simulink model "motor_io_position_GABRIEL"  (R2014b)
settings: Solver=ode1  StartTime=0.0  StopTime=inf  FixedStep=Ts  RelTol=1e-3
PostLoadFcn:
  | , if any(exist('dsrtsu_mdlpostloadfcn', 'file') == [2, 3, 6]), try dsrtsu_mdlpostloadfcn('Execute', bdroot); catch fprintf('Error in PostLoadFcn (dsrtsu_mdlpostloadfcn) for model "%s":\n %s\n', bdroot, lasterr); end, end,
values from neighbouring files (symbols this model uses):
  F_c = 1.5e-3    (= 0.0015)    [continuous_design.m]    (also in workshop1.m)
  F_c_lower = 1.5e-3    (= 0.0015)    [continuous_design.m]    (also in workshop1.m)
  F_c_upper = 1.5e-3    (= 0.0015)    [continuous_design.m]    (also in workshop1.m)
  J1 = 0.0006    [continuous_design.m]    (also in workshop1.m)
  motor = motor_pars    [continuous_design.m]    (also in workshop1.m)
  n = 5    [continuous_design.m]    (also in workshop1.m)
  R_sim = Rd.num{1}    [pbutest.m]
  S_sim = Sd.num{1}    [pbutest.m]
  T_sim = Td.num{1}    [pbutest.m]
  Ts = 2*pi/ws    (= 0.0199466200228)    [continuous_design.m]    (also in pbutest.m = 0.0108705628152; workshop1.m = Ts_p)
libraries: rtilib1104 x5, simulink x1
settings Model: DSRTSU_INTERNAL_RTI_VER=450  DSRTSU_INTERNAL_RTI_TYPE=rti1104  DSRTSU_INTERNAL_RTIFPGA=40  ExtModeArmWhenConnect=off  BufferReuse=off  Creator=user  LastModifiedBy=es2lab2
settings DataIOCC: SignalLoggingSaveFormat=ModelDataLogs  SaveOutput=off  SignalLoggingName=sigsOut
settings OptimizationCC: BlockReduction=off  ConditionallyExecuteInputs=off  OptimizeBlockIOStorage=off  BufferReuse=off  GlobalBufferReuse=off  ExpressionFolding=off  ExpressionDepthLimit=2147483647  LocalBlockOutputs=off  InitFltsAndDblsToZero=on
settings DebuggingCC: SaveWithParameterizedLinksMsg=none  UnderspecifiedInitializationDetection=Classic  MergeDetectMultiDrivingBlocksExec=none  SignalResolutionControl=TryResolveAllWithWarning  SolverPrmCheckMsg=none  MultiTaskDSMMsg=warning  MultiTaskCondExecSysMsg=none  FcnCallInpInsideContextMsg=UseLocalSettings  UnconnectedInputMsg=none  UnconnectedOutputMsg=none  StateNameClashWarn=warning
settings HardwareCC: ProdIntDivRoundTo=Zero  ProdEndianess=BigEndian  ProdHWDeviceType=Generic->Custom  TargetIntDivRoundTo=Zero  TargetEndianess=BigEndian  TargetHWDeviceType=Generic->Custom
settings RTWCC: SystemTargetFile=rti1104.tlc  MakeCommand=make_rti  TemplateMakefile=rti1104.tmf  Description=dSPACE DS1104 Hardware Platform  RetainRTWFile=on  ProcessScript=rti1104_make_rtw_hook  IncludeERTFirstTime=on
settings STFCustomTargetCC: TargetFcnLib=ansi_tfl_tmw.mat  ParMdlRefBuildCompliant=on  GeneratePreprocessorConditionals=Disable all  SystemTargetFile=rti1104.tlc
settings GRTTargetCC: TargetFcnLib=ansi_tfl_tmw.mat  CompOptLevelCompliant=off  ConcurrentExecutionCompliant=off  CombineOutputUpdateFcns=off  MatFileLogging=off  CPPClassGenCompliant=off  GRTInterface=on  ExtModeMexFile=noextcomm

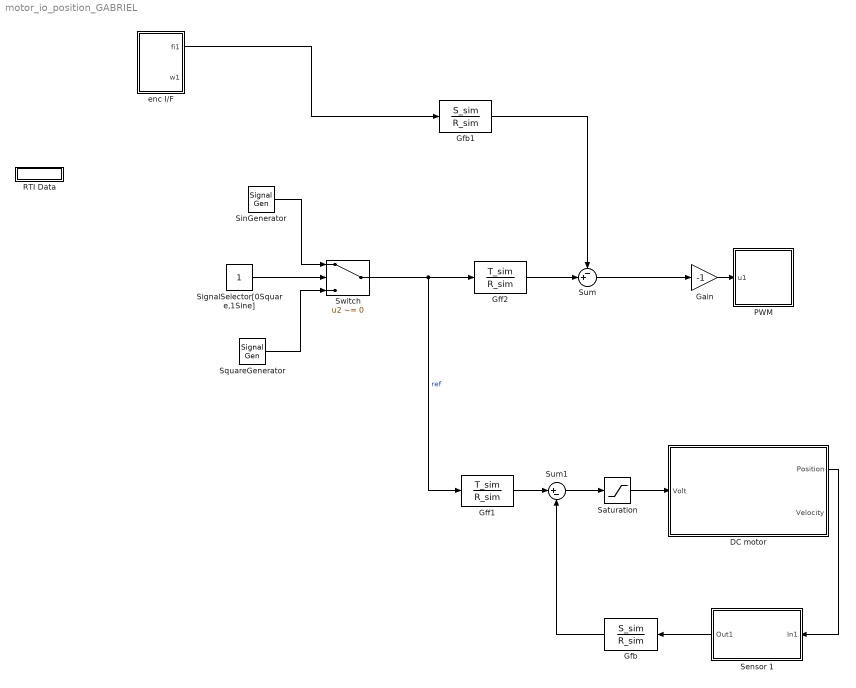
== system motor_io_position_GABRIEL ==
  DC motor : Subsystem
  Gain : Gain  Gain=-1
  Gfb : DiscreteTransferFcn  Numerator=S_sim  Denominator=R_sim  SampleTime=Ts
  Gfb1 : DiscreteTransferFcn  Numerator=S_sim  Denominator=R_sim  SampleTime=Ts
  Gff1 : DiscreteTransferFcn  Numerator=T_sim  Denominator=R_sim  SampleTime=Ts
  Gff2 : DiscreteTransferFcn  Numerator=T_sim  Denominator=R_sim  SampleTime=Ts
  PWM : Subsystem
  RTI Data : Subsystem  Tag=struct('RTIDataServer',struct('RTIDataServerVs','2','RTIModelDescription','struct(''main'',''motor_io_position_GABRIEL'',''sub'',''motor_io_position_GABRIEL'',''isMp'',0)'))  LoadFcn="if exist('rtidc'), try,  rtidc('DataHostBlockClbLoad', gcbh); catch, disp(['Warning: ''LoadFcn'' for RTI Data block failed: ' lasterr]); end, end,"  mask(RTI_DATA_HOST){}
      mask help:
      | RTI Data Block.
      | This block is used by RTI to store internal model-dependent data.
      | Please keep this block on the root level of the model. Deleting this block will result in data loss.
      |
      | NEVER DELETE OR COPY THIS BLOCK!
      settings: CopyFcn="if exist('rtidc'), try,  rtidc('DataHostBlockClbCopy', gcbh); catch, disp(['Warning: ''CopyFcn'' for RTI Data block failed: ' lasterr]); end, end,"  DeleteFcn="if exist('rtidc'), try,  rtidc('DataHostBlockClbDelete', gcbh); catch, disp(['Warning: ''DeleteFcn'' for RTI Data block failed: ' lasterr]); end, end,"  ModelCloseFcn="if exist('rtidc'), try,  rtidc('DataHostBlockClbModelClose', gcbh); catch, disp(['Warning: ''ModelCloseFcn'' for RTI Data block failed: ' lasterr]); end, end,"  PreSaveFcn="if exist('rtidc'), try,  rtidc('DataHostBlockClbPreSave', gcbh); catch, disp(['Warning: ''PreSaveFcn'' for RTI Data block failed: ' lasterr]); end, end,"  PostSaveFcn="if exist('rtidc'), try,  rtidc('DataHostBlockClbPostSave', gcbh); catch, disp(['Warning: ''PostSaveFcn'' for RTI Data block failed: ' lasterr]); end, end,"  NameChangeFcn="if exist('rtidc'), try,  rtidc('DataHostBlockClbNameChange', gcbh); catch, disp(['Warning: ''NameChangeFcn'' for RTI Data block failed: ' lasterr]); end, end,"
      mask Help:
      | RTI Data Block.
      | This block is used by RTI to store internal model-dependent data.
      | Please keep this block on the root level of the model. Deleting this block will result in data loss.
      | 
      | NEVER DELETE OR COPY THIS BLOCK!
      mask Display:
      | text(0.5, 0.5, 'RTI Data', 'HorizontalAlignment', 'center');
      | plot([1 0]);
  Saturation : Saturate  UpperLimit=24  LowerLimit=-24
  Sensor 1 : Subsystem
  SignalSelector[0Square,1Sine] : Constant
  SinGenerator : SignalGenerator  Amplitude=0  Units=rad/sec
  SquareGenerator : SignalGenerator  WaveForm=square  Amplitude=0  Units=rad/sec
  Sum : Sum  Inputs=-+|
  Sum1 : Sum  Inputs=|+-
  Switch : Switch  Criteria=u2 ~= 0
  enc I/F : Subsystem
  wires:
  SinGenerator/1 -> Switch/1
  SquareGenerator/1 -> Switch/3
  SignalSelector[0Square,1Sine]/1 -> Switch/2
  Switch/1 -> Gff1/1, Gff2/1  "ref"
  ? -> ?
  Gain/1 -> PWM/1(u1)
  enc I/F/1(fi1) -> Gfb1/1
  Gfb1/1 -> Sum/1
  Gff2/1 -> Sum/2
  Sum/1 -> Gain/1
  Sensor 1/1(Out1) -> Gfb/1
  DC motor/1(Position) -> Sensor 1/1(In1)
  Saturation/1 -> DC motor/1(Volt)
  Gfb/1 -> Sum1/2
  Sum1/1 -> Saturation/1
  Gff1/1 -> Sum1/1

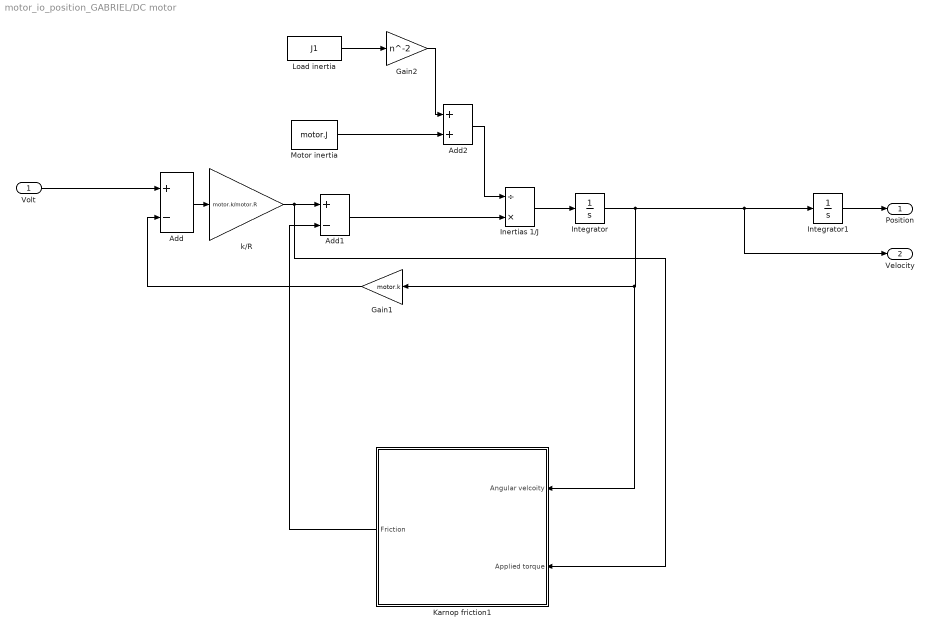
== system motor_io_position_GABRIEL/DC motor ==
  Volt : Inport
  Add : Sum  Inputs=+-
  Add1 : Sum  Inputs=+-
  Add2 : Sum
  Gain1 : Gain  Gain=motor.k
  Gain2 : Gain  Gain=n^-2
  Inertias 1/J : Product  Inputs=/*
  Integrator : Integrator
  Integrator1 : Integrator
  Karnop friction1 : Subsystem
  Load inertia : Constant  Value=J1
  Motor inertia : Constant  Value=motor.J
  "k/R " : Gain  Gain=motor.k/motor.R
  Position : Outport
  Velocity : Outport  Port=2
  wires:
  Add2/1 -> Inertias 1/J/1
  Gain2/1 -> Add2/1
  Load inertia/1 -> Gain2/1
  Motor inertia/1 -> Add2/2
  Integrator/1 -> Integrator1/1, Velocity/1, Gain1/1, Karnop friction1/1(Angular velcoity)
  Volt/1 -> Add/1
  Add1/1 -> Inertias 1/J/2
  Integrator1/1 -> Position/1
  Inertias 1/J/1 -> Integrator/1
  "k/R "/1 -> Add1/1, Karnop friction1/2(Applied torque)
  Add/1 -> "k/R "/1
  Gain1/1 -> Add/2
  Karnop friction1/1(Friction) -> Add1/2

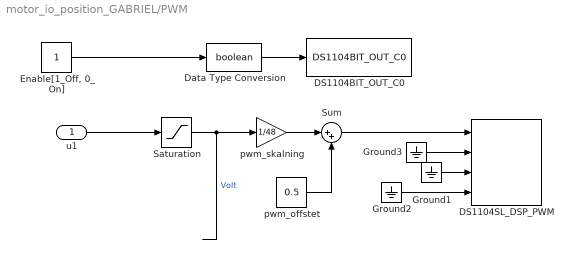
== system motor_io_position_GABRIEL/PWM ==
  u1 : Inport
  DS1104BIT_OUT_C0 : rtilib1104/DS1104 MASTER PPC/DS1104BIT_OUT_C0  ChannelNo=0  InitValue=1  TermMode=0  TermValue=0  Reserved1=[]  Reserved2=[]  Reserved3=[]  Reserved=[]  DialogFcn=gui1104bit_out  UnitName={'DS1104BIT_OUT_C'}  UnitValues={ 0 }  DSProperties=struct('RTI',struct('Version',uint32(1),'BlockType',struct('isSLSource',uint8(0),'isSLSink',uint8(1),'isHWSource',uint8(0),'isHWSink',uint8(1),'isSetup',uint8(0),'isInline',uint8(1),'isNonInline',uint8(0),'isInterrupt',uint8(0),'isChannelwise',uint8(1)),'IOBoardType','DS1104MASTER','UnitType','BIT','Identifier','BITOUTCH','DialogType','ML','BlockSet','NONE','SlaveProcessor','NONE'))
  DS1104SL_DSP_PWM : rtilib1104/DS1104 SLAVE DSP/DS1104SL_DSP_PWM  Parameters=[]  TDef=[]  BoardType=[]  PwmMode=1  Frequency=20000  InitValue=[0.5 0.5 0.5 0.5]  TermMode=[0 0 0 0]  TermValue=[0.5 0.5 0.5 0.5]  Polarity=[1 1 1 1]  DialogFcn=gui1104sl_dsp_pwm  Reserved1=[]  Reserved2=[]  Reserved3=[]  Reserved4=[]  Revision=[]  UnitName={'DS1104SL_DSP_PWM'}  UnitValues={[]}  DSProperties=struct('RTI',struct('Version',uint32(2),'BlockType',struct('isSLSource',uint8(0),'isSLSink',uint8(1),'isHWSource',uint8(0),'isHWSink',uint8(1),'isSetup',uint8(0),'isInline',uint8(1),'isNonInline',uint8(0),'isInterrupt',uint8(0),'isChannelwise',uint8(0)),'IOBoardType','DS1104SLAVE','UnitType','PWM','Identifier','PWM','DialogType','ML','BlockSet','NONE','SlaveProcessor','F240'))  RTIBlockInterface=struct('InputPortsActive',[1 1 1 1],'InputPortsWidth',int32([1 1 1 1]),'InputPortsName',{{['PWM Channel 1'],['PWM Channel 2'],['PWM Channel 3'],['PWM Channel 4']}},'IWork',{{{'',uint32(4)}}},'DialogFcn','rti1104slavepwmgui','InitLevel',1,'BlockDisplay',{{'','auto'}},'IconTransparency','on','MultiSFcn',4,'BlockName',struct('Token',{{'DS1104SL_DSP_PWM'}}))  RTIBlockParameters=struct('PWMSymmetryMode',{{1,'OFF',[]}},'PWMFrequency',{{'50000','OFF',[]}},'PWMPolarityMode',{{[1 1 1 1 1],'OFF',[]}},'ChannelNo',{{[1 2 3 4],'OFF',[]}},'SuspendModeInit',{{[0 0 0 0 1],'OFF',[]}},'TTLModeInit',{{[2 2 2 2 2],'OFF',[]}},'DutyCycleInitValueCh1',{{'0.5','OFF',[]}},'DutyCycleInitValueCh2',{{'0.5','OFF',[]}},'DutyCycleInitValueCh3',{{'0.5','OFF',[]}},'DutyCycleInitValueCh4',{{'0.5','OFF',[]}},'DutyCycleInitValueCh5',{{'0.5','OFF',[]}},'EnablePWMStop',{{[0 0 0 0 0],'OFF',[]}},'SuspendModeTerm',{{[0 0 0 0 1],'OFF',[]}},'TTLModeTerm',{{[2 2 2 2 2],'OFF',[]}},'DutyCycleTermValueCh1',{{'0.5','OFF',[]}},'DutyCycleTermValueCh2',{{'0.5','OFF',[]}},'DutyCycleTermValueCh3',{{'0.5','OFF',[]}},'DutyCycleTermValueCh4',{{'0.5','OFF',[]}},'DutyCycleTermValueCh5',{{'0.5','OFF',[]}},'TLCFileName',{{'rti1104pwm','OFF',[]}})  RTISFcnParameters=struct('PWMSymmetryMode','double','PWMFrequency','double','PWMPolarityMode','double','ChannelNo','double','SuspendModeInit','double','TTLModeInit','double','DutyCycleInitValueCh1','double','DutyCycleInitValueCh2','double','DutyCycleInitValueCh3','double','DutyCycleInitValueCh4','double','EnablePWMStop','double','SuspendModeTerm','double','TTLModeTerm','double','DutyCycleTermValueCh1','double','DutyCycleTermValueCh2','double','DutyCycleTermValueCh3','double','DutyCycleTermValueCh4','double','TLCFileName','char')  RTIBlockParaDefault=struct('PWMSymmetryMode',1,'PWMFrequency',100,'PWMPolarityMode',[1 1 1 1 1],'ChannelNo',[1 2 3 4],'SuspendModeInit',[1 1 1 1 1],'TTLModeInit',[2 2 2 2 2],'DutyCycleInitValueCh1',0.5,'DutyCycleInitValueCh2',0.5,'DutyCycleInitValueCh3',0.5,'DutyCycleInitValueCh4',0.5,'DutyCycleInitValueCh5',0.5,'EnablePWMStop',[1 1 1 1 0],'SuspendModeTerm',[1 1 1 1 1],'TTLModeTerm',[2 2 2 2 2],'DutyCycleTermValueCh1',0.5,'DutyCycleTermValueCh2',0.5,'DutyCycleTermValueCh3',0.5,'DutyCycleTermValueCh4',0.5,'DutyCycleTermValueCh5',0.5,'TLCFileName','rti1104pwm')
  Data Type Conversion : DataTypeConversion  OutDataTypeStr=boolean  SaturateOnIntegerOverflow=on  RndMeth=Zero
  "Enable[1_Off, 0_On]" : Constant
  Ground1 : Ground
  Ground2 : Ground
  Ground3 : Ground
  Saturation : Saturate  UpperLimit=24  LowerLimit=-24
  Sum : Sum  Inputs=|++  SaturateOnIntegerOverflow=on
  pwm_offstet : Constant  Value=0.5
  pwm_skalning : Gain  Gain=1/48  SaturateOnIntegerOverflow=on  OutDataTypeStr=Inherit: Same as input  ParamDataTypeStr=Inherit: Same as input
  wires:
  "Enable[1_Off, 0_On]"/1 -> Data Type Conversion/1
  Data Type Conversion/1 -> DS1104BIT_OUT_C0/1
  pwm_skalning/1 -> Sum/1
  Sum/1 -> DS1104SL_DSP_PWM/1
  pwm_offstet/1 -> Sum/2
  u1/1 -> Saturation/1
  Ground1/1 -> DS1104SL_DSP_PWM/3
  Ground2/1 -> DS1104SL_DSP_PWM/4
  Ground3/1 -> DS1104SL_DSP_PWM/2
  Saturation/1 -> pwm_skalning/1  "Volt"

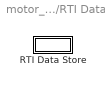
== system motor_io_position_GABRIEL/RTI Data ==
  RTI Data Store : Subsystem  Tag=struct('private',struct('version',struct('dsVer',uint32(2)),'access',struct('modified',['06-Apr-2016 18:22:15'],'type','Model','isPerm',1)))  mask(RTI_DATA_STORE){}
      mask help:
      | RTI Data Store Block. This block is used by RTI to store internal model dependent data. Deleting this block will result in data loss.
      |
      | NEVER DELETE, COPY, OR MODIFY THIS BLOCK!
      mask Help:
      | RTI Data Store Block. This block is used by RTI to store internal model dependent data. Deleting this block will result in data loss.
      | 
      | NEVER DELETE, COPY, OR MODIFY THIS BLOCK!
      mask Display: text(0.5, 0.5, ' ', 'HorizontalAlignment', 'center');

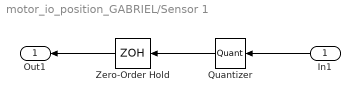
== system motor_io_position_GABRIEL/Sensor 1 ==
  In1 : Inport
  Quantizer : Quantizer  QuantizationInterval=quant
  Zero-Order Hold : ZeroOrderHold  SampleTime=Ts
  Out1 : Outport
  wires:
  Quantizer/1 -> Zero-Order Hold/1
  In1/1 -> Quantizer/1
  Zero-Order Hold/1 -> Out1/1

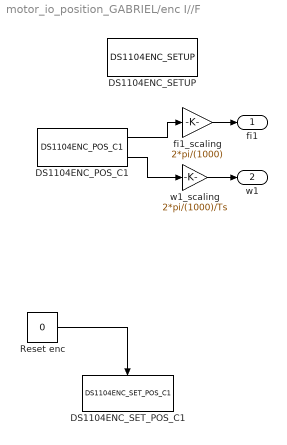
== system motor_io_position_GABRIEL/enc I//F ==
  DS1104ENC_POS_C1 : rtilib1104/DS1104 MASTER PPC/DS1104ENC_POS_C1  ChannelNo=1  PosValue=0  Reserved1=[]  Reserved2=[]  Reserved3=[]  Reserved4=[]  DialogFcn=gui1104enc_pos  UnitName={'DS1104ENC_POS_C'}  UnitValues={ 1 }  DSProperties=struct('RTI',struct('Version',uint32(1),'BlockType',struct('isSLSource',uint8(1),'isSLSink',uint8(0),'isHWSource',uint8(1),'isHWSink',uint8(0),'isSetup',uint8(0),'isInline',uint8(1),'isNonInline',uint8(0),'isInterrupt',uint8(0),'isChannelwise',uint8(1)),'IOBoardType','DS1104MASTER','UnitType','ENC','Identifier','ENCPOSCH','DialogType','ML','BlockSet','NONE','SlaveProcessor','NONE'))
  DS1104ENC_SETUP : rtilib1104/DS1104 MASTER PPC/DS1104ENC_SETUP  Reserved1=[]  Reserved2=[]  Reserved3=[]  Reserved4=[]  DialogFcn=gui1104enc_setup  UnitName={'DS1104ENC_SETUP'}  UnitValues={ [] }  DSProperties=struct('RTI',struct('Version',uint32(1),'BlockType',struct('isSLSource',uint8(0),'isSLSink',uint8(0),'isHWSource',uint8(0),'isHWSink',uint8(0),'isSetup',uint8(0),'isInline',uint8(1),'isNonInline',uint8(0),'isInterrupt',uint8(0),'isChannelwise',uint8(0)),'IOBoardType','DS1104MASTER','UnitType','ENC','Identifier','ENCSETUP','DialogType','ML','BlockSet','NONE','SlaveProcessor','NONE'))
      settings: SignalType=[1 0]
  DS1104ENC_SET_POS_C1 : rtilib1104/DS1104 MASTER PPC/DS1104ENC_SET_POS_C1  ChannelNo=1  PosValue=0  Reserved1=[]  Reserved2=[]  Reserved3=[]  Reserved4=[]  DialogFcn=gui1104enc_set_pos  UnitName={'DS1104ENC_SET_POS_C'}  UnitValues={ 1 }  DSProperties=struct('RTI',struct('Version',uint32(1),'BlockType',struct('isSLSource',uint8(0),'isSLSink',uint8(1),'isHWSource',uint8(0),'isHWSink',uint8(1),'isSetup',uint8(0),'isInline',uint8(1),'isNonInline',uint8(0),'isInterrupt',uint8(0),'isChannelwise',uint8(1)),'IOBoardType','DS1104MASTER','UnitType','ENC','Identifier','ENCRESET','DialogType','ML','BlockSet','NONE','SlaveProcessor','NONE'))
  Reset enc : Constant  Value=0
  fi1_scaling : Gain  Gain=2*pi/(1000)  SaturateOnIntegerOverflow=on  OutDataTypeStr=Inherit: Same as input  ParamDataTypeStr=Inherit: Same as input
  w1_scaling : Gain  Gain=2*pi/(1000)/Ts  SaturateOnIntegerOverflow=on  OutDataTypeStr=Inherit: Same as input  ParamDataTypeStr=Inherit: Same as input
  fi1 : Outport
  w1 : Outport  Port=2
  wires:
  Reset enc/1 -> DS1104ENC_SET_POS_C1/Trigger
  DS1104ENC_POS_C1/1 -> fi1_scaling/1
  DS1104ENC_POS_C1/2 -> w1_scaling/1
  fi1_scaling/1 -> fi1/1
  w1_scaling/1 -> w1/1

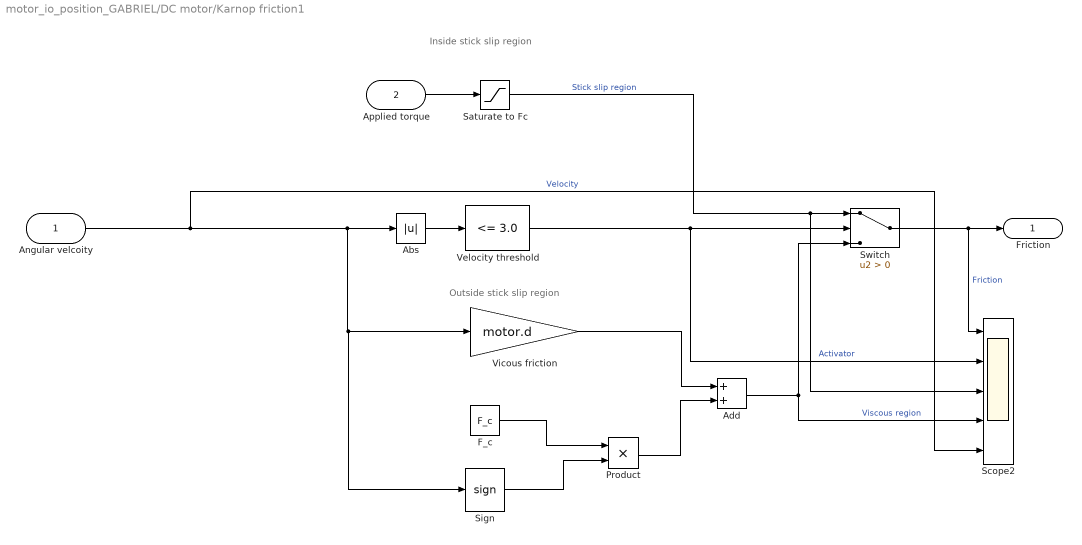
== system motor_io_position_GABRIEL/DC motor/Karnop friction1 ==
  note: Outside stick slip region
  note: Inside stick slip region
  Angular velcoity : Inport
  Applied torque : Inport  Port=2
  Abs : Abs  ZeroCross=off
  Add : Sum
  F_c : Constant  Value=F_c
  Product : Product
  Saturate to Fc : Saturate  UpperLimit=F_c_upper  LowerLimit=-F_c_lower  ZeroCross=off
  Scope2 : Scope  NumInputPorts=5
      settings: ShowLegends=on  YMin=-0.00177~-0.125~0.0009~-0.00177~-138.1533~-0.12501~-0.12501~-0.12501  YMax=0.00177~1.125~0.0011~0.00177~138.10681~0.12501~0.12501~0.12501  SaveName=ScopeData3
  Sign : Signum  ZeroCross=off
  Switch : Switch  Criteria=u2 > Threshold  ZeroCross=off
  "Velocity threshold " : simulink/Logic and Bit Operations/Compare To Constant  relop=<=  const=3.0  OutDataTypeStr=boolean
  Vicous friction : Gain  Gain=motor.d
  Friction : Outport
  wires:
  Applied torque/1 -> Saturate to Fc/1
  Add/1 -> Scope2/4, Switch/3  "Viscous region"
  Sign/1 -> Product/2
  F_c/1 -> Product/1
  Vicous friction/1 -> Add/1
  Product/1 -> Add/2
  Abs/1 -> "Velocity threshold "/1
  "Velocity threshold "/1 -> Switch/2, Scope2/2  "Activator"
  Angular velcoity/1 -> Sign/1, Vicous friction/1, Abs/1, Scope2/5  "Velocity"
  Switch/1 -> Friction/1, Scope2/1  "Friction"
  Saturate to Fc/1 -> Switch/1, Scope2/3  "Stick slip region"

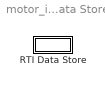
== system motor_io_position_GABRIEL/RTI Data/RTI Data Store ==
  RTI Data Store : Subsystem  mask(RTI_DATA_STORE){}
      mask help:
      | RTI Data Store Block. This block is used by RTI to store internal model dependent data. Deleting this block will result in data loss.
      |
      | NEVER DELETE, COPY, OR MODIFY THIS BLOCK!
      mask Help:
      | RTI Data Store Block. This block is used by RTI to store internal model dependent data. Deleting this block will result in data loss.
      | 
      | NEVER DELETE, COPY, OR MODIFY THIS BLOCK!
      mask Display: text(0.5, 0.5, ' ', 'HorizontalAlignment', 'center');

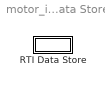
== system motor_io_position_GABRIEL/RTI Data/RTI Data Store/RTI Data Store ==
  RTI Data Store : Subsystem  mask(RTI_DATA_STORE){}
      mask help:
      | RTI Data Store Block. This block is used by RTI to store internal model dependent data. Deleting this block will result in data loss.
      |
      | NEVER DELETE, COPY, OR MODIFY THIS BLOCK!
      mask Help:
      | RTI Data Store Block. This block is used by RTI to store internal model dependent data. Deleting this block will result in data loss.
      | 
      | NEVER DELETE, COPY, OR MODIFY THIS BLOCK!
      mask Display: text(0.5, 0.5, ' ', 'HorizontalAlignment', 'center');

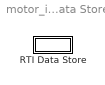
== system motor_io_position_GABRIEL/RTI Data/RTI Data Store/RTI Data Store/RTI Data Store ==
  RTI Data Store : Subsystem  mask(RTI_DATA_STORE){}
      mask help:
      | RTI Data Store Block. This block is used by RTI to store internal model dependent data. Deleting this block will result in data loss.
      |
      | NEVER DELETE, COPY, OR MODIFY THIS BLOCK!
      mask Help:
      | RTI Data Store Block. This block is used by RTI to store internal model dependent data. Deleting this block will result in data loss.
      | 
      | NEVER DELETE, COPY, OR MODIFY THIS BLOCK!
      mask Display: text(0.5, 0.5, ' ', 'HorizontalAlignment', 'center');

== system motor_io_position_GABRIEL/RTI Data/RTI Data Store/RTI Data Store/RTI Data Store/RTI Data Store ==
